simulink model "test_fix"  (R2023b)
settings: Solver=FixedStepDiscrete  StartTime=0.0  StopTime=inf  RelTol=1e-3  EnableMultiTasking=on
libraries: LSL x1, Tools x1
settings Model: Creator=uceerjp  LastModifiedBy=uceerjp
settings SolverCC: AlgebraicLoopSolver=TrustRegion  AutoInsertRateTranBlk=on
settings DataIOCC: LimitDataPoints=on  SaveFormat=Array  ReturnWorkspaceOutputs=off
settings OptimizationCC: LifeSpan=inf
settings DebuggingCC: UnconnectedInputMsg=warning  UnconnectedOutputMsg=warning  UnconnectedLineMsg=warning  FrameProcessingCompatibilityMsg=none  SFUnexpectedBacktrackingDiag=warning  SFNoUnconditionalDefaultTransitionDiag=warning  SFExecutionAtInitializationDiag=none  ArithmeticOperatorsInVariantConditions=warning
settings HardwareCC: ProdBitPerPointer=32  ProdBitPerSizeT=32  ProdBitPerPtrDiffT=32  ProdLargestAtomicFloat=None  ProdIntDivRoundTo=Undefined  ProdEndianess=Unspecified  ProdWordSize=32  ProdHWDeviceType=32-bit Generic
settings ModelReferenceCC: EnableRefExpFcnMdlSchedulingChecks=on  PropagateSignalLabelsOutOfModel=off
settings SFSimCC: SimUseLocalCustomCode=off  CustomCodeUndefinedFunction=UseInterfaceOnly
settings RTWCC: RTWUseLocalCustomCode=off
settings CodeAppCC: StateflowObjectComments=on
settings GRTTargetCC: TargetLangStandard=C89/C90 (ANSI)
settings ConfigComp: CovMetricSettings=dw  CovSaveCumulativeToWorkspaceVar=on  CovSaveSingleToWorkspaceVar=on  CovExternalEMLEnable=off

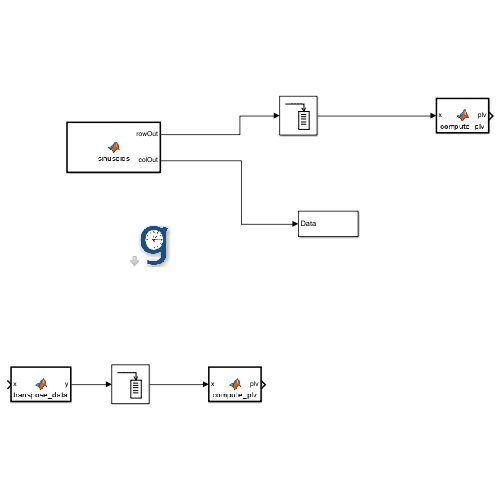
[thumbnail: Simulink's stored preview of the top-level diagram]
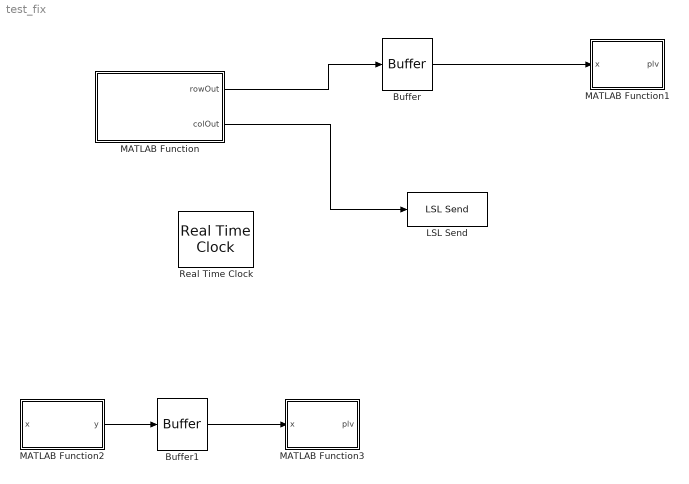
== system test_fix ==
  Buffer : Buffer  N=768  V=640  OutputFrames=off
  Buffer1 : Buffer  N=256  V=128  OutputFrames=off
  LSL Send : LSL/LSL Send  noChannels=62  lslPropName='gtec'  lslPropValue='EEG'  sampleRate=256
      settings: SourceProductName=g.HIsys
  MATLAB Function : MATLAB Function  TreatAsAtomicUnit=on  SystemSampleTime=0.00390625
  MATLAB Function1 : MATLAB Function  TreatAsAtomicUnit=on  SystemSampleTime=0.00390625
  MATLAB Function2 : MATLAB Function  TreatAsAtomicUnit=on  SystemSampleTime=0.00390625
  MATLAB Function3 : MATLAB Function  TreatAsAtomicUnit=on  SystemSampleTime=0.00390625
  Real Time Clock : Tools/Real Time Clock  timeprofile=off
      settings: SourceProductName=g.HIsys
  wires:
  MATLAB Function/1(rowOut) -> Buffer/1
  Buffer/1 -> MATLAB Function1/1(x)
  MATLAB Function/2(colOut) -> LSL Send/1
  MATLAB Function2/1(y) -> Buffer1/1
  Buffer1/1 -> MATLAB Function3/1(x)

== matlab function test_fix/MATLAB Function ==
  data: rowOut output; colOut output
function [rowOut, colOut] = sinusoids()
% Outputs:
%   rowOut → [1×62] for Buffer and PLV processing
%   colOut → [62×1] for LSL streaming

persistent t amps freqs_base freq_mod_phase phase_base shared_noise_phase
dt = 1/256;

if isempty(t)
    t = 0;
    rng(42);  % Reproducibility

    amps = 0.5 + rand(1,62)*1.5;          % amplitudes: 0.5–2.0
    freqs_base = 4 + rand(1,62)*36;       % base frequencies: 4–40 Hz
    freq_mod_phase = rand(1,62)*2*pi;     % modulation phase offsets
    phase_base = rand(1,62)*2*pi;         % base phases
    shared_noise_phase = 2*pi*rand();     % for correlated noise
end

% Dynamic frequency modulation (adds time variation)
mod_freq = 0.7;  % Hz
freqs = freqs_base + 5 * sin(2*pi*mod_freq*t + freq_mod_phase);
omega = 2*pi*freqs;
instant_phase = omega*t + phase_base;

% Shared low-frequency noise across all channels
shared_noise = 0.2 * sin(2*pi*0.5*t + shared_noise_phase) + 0.05*randn();

% Generate raw sinusoidal signals
signal = amps .* sin(instant_phase);

% Add shared noise
signal = signal + shared_noise;

% Format outputs
rowOut = reshape(signal, 1, 62);  % for Buffer block (row vector)
colOut = reshape(signal, 62, 1);  % for LSL streaming (column vector)

% Advance time
t = t + dt;

== matlab function test_fix/MATLAB Function2 ==
  data: x input; y output
function y = transpose_data(x)
% Flip dimensions so PLV function receives channels x samples
y = x';
end

== matlab function test_fix/MATLAB Function3 ==
  data: plv output; x input
function plv = compute_plv(x)
% Input x: [256 × 62], output: [62 × 62]

x = x';  % Now [62 × 256]
N = size(x,1);
plv = zeros(N);

phases = angle(hilbert(x')');  % Hilbert across time

for i = 1:N
    for j = 1:N
        if i ~= j
            dphi = phases(i,:) - phases(j,:);
            plv(i,j) = abs(mean(exp(1i * dphi)));
        else
            plv(i,j) = 0;
        end
    end
end

imagesc(plv, [0 1]);
axis([0 N 0 N]);
axis square;
drawnow;

== matlab function test_fix/MATLAB Function1 ==
  data: plv output; x input
function plv = compute_plv(x)
% Input x: [256 × 62], output: [62 × 62]

x = x';  % Now [62 × 256]
N = size(x,1);
plv = zeros(N);

phases = angle(hilbert(x')');  % Hilbert across time

for i = 1:N
    for j = 1:N
        if i ~= j
            dphi = phases(i,:) - phases(j,:);
            plv(i,j) = abs(mean(exp(1i * dphi)));
        else
            plv(i,j) = 0;
        end
    end
end

imagesc(plv, [0 1]);
axis([0.5 N+0.5 0.5 N+0.5]);
axis square;
drawnow;
